simulink model "modern_kontrol_elmas"  (R2024a)
settings: Solver=VariableStepAuto  StartTime=0.0  StopTime=2.5  RelTol=1e-3
values from neighbouring files (symbols this model uses):
  kazanc = 0.98    [modern_kontrol_5.m]
  T = 1/(kt*min_kok)    [modern_kontrol_5.m]
  to = 115e-3    (= 0.115)    [modern_kontrol_5.m]
libraries: simulink_extras x1
settings Model: Creator=ireme  LastModifiedBy=ESMA
settings RTWCC: GPUComputeCapability=3.5

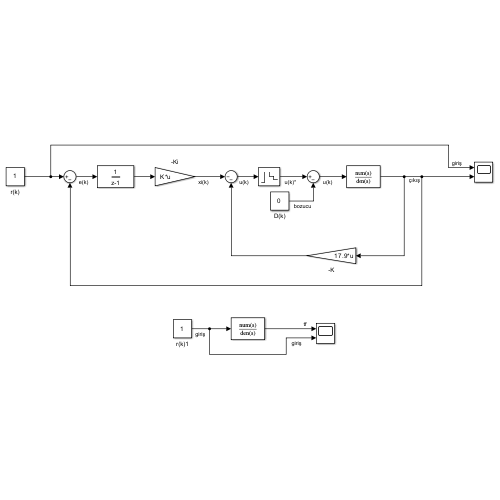
[thumbnail: Simulink's stored preview of the top-level diagram]
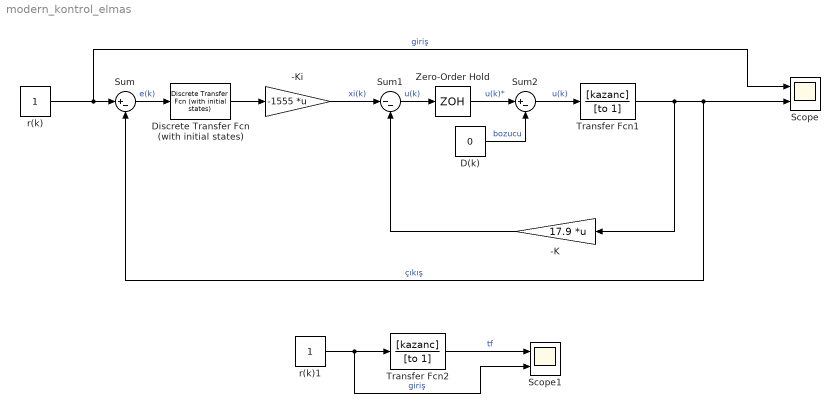
== system modern_kontrol_elmas ==
  -K : Gain  Gain=17.9  Multiplication=Matrix(K*u)
  -Ki : Gain  Gain=-1555  Multiplication=Matrix(K*u)
  D(k) : Constant  Value=0  SampleTime=T
  Discrete Transfer Fcn (with initial states) : simulink_extras/Additional Discrete/Discrete Transfer Fcn (with initial states)  N=[1]  D="[1  -1]"  X0=0  TS=T
  Scope : Scope  NumInputPorts=2
  Scope1 : Scope  NumInputPorts=2
  Sum : Sum  Inputs=|+-
  Sum1 : Sum  Inputs=|--
  Sum2 : Sum  Inputs=|+-
  Transfer Fcn1 : TransferFcn  Numerator=[kazanc]  Denominator=[to 1]
  Transfer Fcn2 : TransferFcn  Numerator=[kazanc]  Denominator=[to 1]
  Zero-Order Hold : ZeroOrderHold  SampleTime=T
  r(k) : Constant
  r(k)1 : Constant
  wires:
  -K/1 -> Sum1/2
  Transfer Fcn1/1 -> -K/1, Scope/2, Sum/2  "çıkış"
  Sum2/1 -> Transfer Fcn1/1  "u(k)"
  D(k)/1 -> Sum2/2  "bozucu"
  Zero-Order Hold/1 -> Sum2/1  "u(k)*"
  -Ki/1 -> Sum1/1  "xi(k)"
  Sum1/1 -> Zero-Order Hold/1  "u(k)"
  Discrete Transfer Fcn (with initial states)/1 -> -Ki/1
  Sum/1 -> Discrete Transfer Fcn (with initial states)/1  "e(k)"
  r(k)/1 -> Sum/1, Scope/1  "giriş"
  Transfer Fcn2/1 -> Scope1/1  "tf"
  r(k)1/1 -> Transfer Fcn2/1, Scope1/2  "giriş"
